simulink library "libbha_parameters"  (R2015b)
settings: Solver=FixedStepDiscrete  StartTime=0.0  StopTime=Inf  FixedStep=0.004  RelTol=1e-3
PostLoadFcn:
  | , if any(exist('dsrtsu_mdlpostloadfcn', 'file') == [2, 3, 6]), try dsrtsu_mdlpostloadfcn('Execute', bdroot); catch fprintf('Error in PostLoadFcn (dsrtsu_mdlpostloadfcn) for model "%s":\n %s\n', bdroot, lasterr); end, end,
undefined symbols (not defined in the file or in its folder): BHA, CONST
libraries: libbha_kinematic x12
(part 2 of 2)

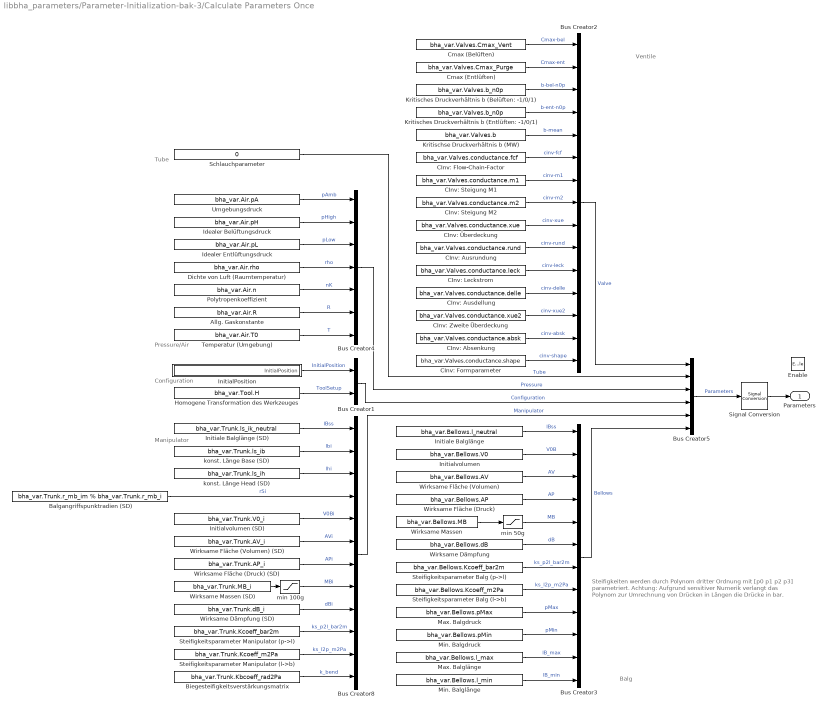
== system libbha_parameters/Parameter-Initialization-bak-3/Calculate Parameters Once ==
  note: Tube
  note: Pressure/Air
  note: Configuration
  note: Manipulator
  note: Ventile
  note: Balg
  note: Steifigkeiten werden durch Polynom dritter Ordnung mit [p0 p1 p2 p3]
      | parametriert. Achtung: Aufgrund sensitiver Numerik verlangt das Polynom
      | zur Umrechnung von Drücken in Längen die Drücke in bar.
  Enable : EnablePort  PropagateVarSize=During execution
  Allg. Gaskonstante : Constant  Value=bha_var.Air.R
  Balgangriffspunktradien (SD) : Constant  Value=bha_var.Trunk.r_mb_im % bha_var.Trunk.r_mb_i
      settings: AttributesFormatString=|
      | Radien Manipulator-Balg
      | r_mb_im: am Sektionskopf
      | r_mb_i:    an Sektionsmitte
  Biegesteifigkeitsverstärkungsmatrix : Constant  Value=bha_var.Trunk.Kbcoeff_rad2Pa
  Bus Creator1 : BusCreator  Inputs=2
  Bus Creator3 : BusCreator  Inputs=12
  Bus Creator4 : BusCreator  Inputs=7
  Bus Creator8 : BusCreator  Inputs=12
  Bus Creator2 : BusCreator  Inputs=15
  Bus Creator5 : BusCreator  Inputs=6
  CInv: Absenkung : Constant  Value=bha_var.Valves.conductance.absk
  CInv: Ausdellung : Constant  Value=bha_var.Valves.conductance.delle
  CInv: Ausrundung : Constant  Value=bha_var.Valves.conductance.rund
  CInv: Flow-Chain-Factor : Constant  Value=bha_var.Valves.conductance.fcf
  CInv: Formparameter : Constant  Value=bha_var.Valves.conductance.shape
  CInv: Leckstrom : Constant  Value=bha_var.Valves.conductance.leck
  CInv: Steigung M1 : Constant  Value=bha_var.Valves.conductance.m1
  CInv: Steigung M2 : Constant  Value=bha_var.Valves.conductance.m2
  CInv: Zweite Überdeckung : Constant  Value=bha_var.Valves.conductance.xue2
  CInv: Überdeckung : Constant  Value=bha_var.Valves.conductance.xue
  Cmax (Belüften) : Constant  Value=bha_var.Valves.Cmax_Vent
  Cmax (Entlüften) : Constant  Value=bha_var.Valves.Cmax_Purge
  Dichte von Luft (Raumtemperatur) : Constant  Value=bha_var.Air.rho
  Homogene Transformation des Werkzeuges : Constant  Value=bha_var.Tool.H
  Idealer Belüftungsdruck : Constant  Value=bha_var.Air.pH
  Idealer Entlüftungsdruck : Constant  Value=bha_var.Air.pL
  InitialPosition : Subsystem
  Initiale Balglänge : Constant  Value=bha_var.Bellows.l_neutral
  Initiale Balglänge (SD) : Constant  Value=bha_var.Trunk.ls_ik_neutral
  Initialvolumen : Constant  Value=bha_var.Bellows.V0
  Initialvolumen (SD) : Constant  Value=bha_var.Trunk.V0_i
  Kritisches Druckverhältnis b (Belüften: -1/0/1) : Constant  Value=bha_var.Valves.b_n0p
  Kritisches Druckverhältnis b (Entlüften: -1/0/1) : Constant  Value=bha_var.Valves.b_n0p
  Kritischse Druckverhältnis b (MW) : Constant  Value=bha_var.Valves.b
  Max. Balgdruck : Constant  Value=bha_var.Bellows.pMax
  Max. Balglänge : Constant  Value=bha_var.Bellows.l_max
  Min. Balgdruck : Constant  Value=bha_var.Bellows.pMin
  Min. Balglänge : Constant  Value=bha_var.Bellows.l_min
  Polytropenkoeffizient : Constant  Value=bha_var.Air.n
  Schlauchparameter : Constant  Value=0
  Signal Conversion : SignalConversion
  Steifigkeitsparameter Balg (l->b) : Constant  Value=bha_var.Bellows.Kcoeff_m2Pa
  Steifigkeitsparameter Balg (p->l) : Constant  Value=bha_var.Bellows.Kcoeff_bar2m
  Steifigkeitsparameter Manipulator (l->b) : Constant  Value=bha_var.Trunk.Kcoeff_m2Pa
  Steifigkeitsparameter Manipulator (p->l) : Constant  Value=bha_var.Trunk.Kcoeff_bar2m
  Temperatur (Umgebung) : Constant  Value=bha_var.Air.T0
  Umgebungsdruck : Constant  Value=bha_var.Air.pA
  Wirksame Dämpfung : Constant  Value=bha_var.Bellows.dB
  Wirksame Dämpfung (SD) : Constant  Value=bha_var.Trunk.dB_i
  Wirksame Fläche (Druck) : Constant  Value=bha_var.Bellows.AP
  Wirksame Fläche (Druck) (SD) : Constant  Value=bha_var.Trunk.AP_i
  Wirksame Fläche (Volumen) : Constant  Value=bha_var.Bellows.AV
  Wirksame Fläche (Volumen) (SD) : Constant  Value=bha_var.Trunk.AV_i
  Wirksame Massen : Constant  Value=bha_var.Bellows.MB
  Wirksame Massen (SD) : Constant  Value=bha_var.Trunk.MB_i
  konst. Länge Base (SD) : Constant  Value=bha_var.Trunk.ls_ib
  konst. Länge Head (SD) : Constant  Value=bha_var.Trunk.ls_ih
  min 100g : Saturate  UpperLimit=inf  LowerLimit=0.1
  min 50g : Saturate  UpperLimit=inf  LowerLimit=0.1
  Parameters : Outport
  wires:
  CInv: Zweite Überdeckung/1 -> Bus Creator2/13  "cinv-xue2"
  CInv: Ausdellung/1 -> Bus Creator2/12  "cinv-delle"
  CInv: Formparameter/1 -> Bus Creator2/15  "cinv-shape"
  CInv: Absenkung/1 -> Bus Creator2/14  "cinv-absk"
  Kritischse Druckverhältnis b (MW)/1 -> Bus Creator2/5  "b-mean"
  Schlauchparameter/1 -> Bus Creator5/2  "Tube"
  Biegesteifigkeitsverstärkungsmatrix/1 -> Bus Creator8/12  "k_bend"
  Steifigkeitsparameter Manipulator (p->l)/1 -> Bus Creator8/10  "ks_p2l_bar2m"
  Steifigkeitsparameter Manipulator (l->b)/1 -> Bus Creator8/11  "ks_l2p_m2Pa"
  Bus Creator5/1 -> Signal Conversion/1  "Parameters"
  Wirksame Massen/1 -> min 50g/1
  Wirksame Massen (SD)/1 -> min 100g/1
  Umgebungsdruck/1 -> Bus Creator4/1  "pAmb"
  Initiale Balglänge/1 -> Bus Creator3/1  "lBss"
  Wirksame Fläche (Druck)/1 -> Bus Creator3/4  "AP"
  Bus Creator8/1 -> Bus Creator5/5  "Manipulator"
  min 100g/1 -> Bus Creator8/8  "MBi"
  Bus Creator3/1 -> Bus Creator5/6  "Bellows"
  Initialvolumen (SD)/1 -> Bus Creator8/5  "V0Bi"
  Wirksame Dämpfung (SD)/1 -> Bus Creator8/9  "dBi"
  Homogene Transformation des Werkzeuges/1 -> Bus Creator1/2  "ToolSetup"
  Wirksame Fläche (Druck) (SD)/1 -> Bus Creator8/7  "APi"
  Wirksame Fläche (Volumen) (SD)/1 -> Bus Creator8/6  "AVi"
  Initialvolumen/1 -> Bus Creator3/2  "V0B"
  Steifigkeitsparameter Balg (p->l)/1 -> Bus Creator3/7  "ks_p2l_bar2m"
  konst. Länge Head (SD)/1 -> Bus Creator8/3  "lhi"
  konst. Länge Base (SD)/1 -> Bus Creator8/2  "lbi"
  Balgangriffspunktradien (SD)/1 -> Bus Creator8/4  "rSi"
  min 50g/1 -> Bus Creator3/5  "MB"
  Wirksame Dämpfung/1 -> Bus Creator3/6  "dB"
  Dichte von Luft (Raumtemperatur)/1 -> Bus Creator4/4  "rho"
  Temperatur (Umgebung)/1 -> Bus Creator4/7  "T"
  Idealer Entlüftungsdruck/1 -> Bus Creator4/3  "pLow"
  Wirksame Fläche (Volumen)/1 -> Bus Creator3/3  "AV"
  Bus Creator2/1 -> Bus Creator5/1  "Valve"
  Polytropenkoeffizient/1 -> Bus Creator4/5  "nK"
  Allg. Gaskonstante/1 -> Bus Creator4/6  "R"
  InitialPosition/1(InitialPosition) -> Bus Creator1/1  "InitialPosition"
  Steifigkeitsparameter Balg (l->b)/1 -> Bus Creator3/8  "ks_l2p_m2Pa"
  Bus Creator4/1 -> Bus Creator5/3  "Pressure"
  Initiale Balglänge (SD)/1 -> Bus Creator8/1  "lBss"
  Bus Creator1/1 -> Bus Creator5/4  "Configuration"
  Signal Conversion/1 -> Parameters/1
  Idealer Belüftungsdruck/1 -> Bus Creator4/2  "pHigh"
  Kritisches Druckverhältnis b (Belüften: -1/0/1)/1 -> Bus Creator2/3  "b-bel-n0p"
  Cmax (Belüften)/1 -> Bus Creator2/1  "Cmax-bel"
  Cmax (Entlüften)/1 -> Bus Creator2/2  "Cmax-ent"
  Kritisches Druckverhältnis b (Entlüften: -1/0/1)/1 -> Bus Creator2/4  "b-ent-n0p"
  CInv: Leckstrom/1 -> Bus Creator2/11  "cinv-leck"
  CInv: Ausrundung/1 -> Bus Creator2/10  "cinv-rund"
  CInv: Überdeckung/1 -> Bus Creator2/9  "cinv-xue"
  CInv: Steigung M2/1 -> Bus Creator2/8  "cinv-m2"
  CInv: Steigung M1/1 -> Bus Creator2/7  "cinv-m1"
  CInv: Flow-Chain-Factor/1 -> Bus Creator2/6  "cinv-fcf"
  Max. Balgdruck/1 -> Bus Creator3/9  "pMax"
  Min. Balgdruck/1 -> Bus Creator3/10  "pMin"
  Max. Balglänge/1 -> Bus Creator3/11  "lB_max"
  Min. Balglänge/1 -> Bus Creator3/12  "lB_min"

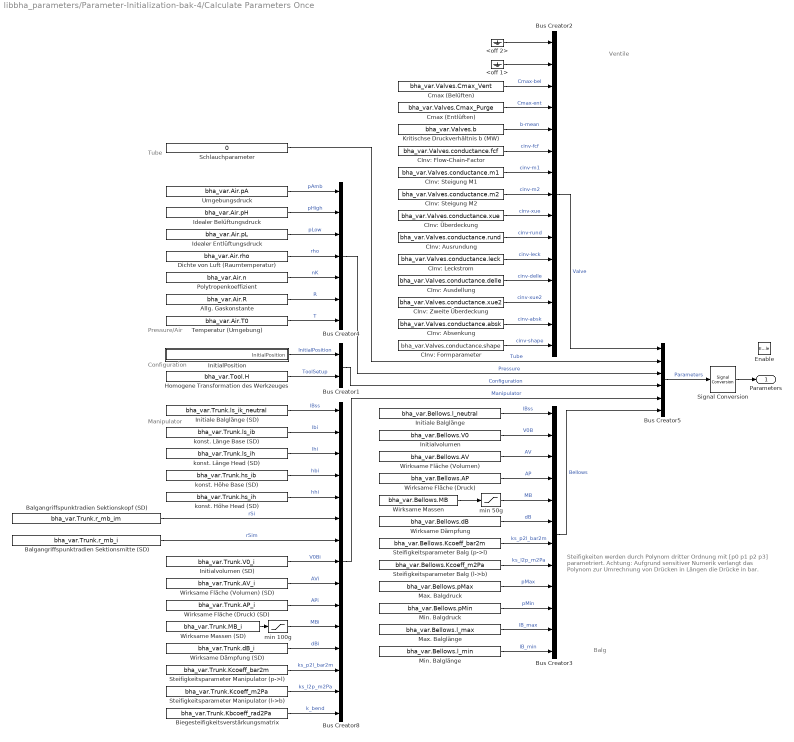
== system libbha_parameters/Parameter-Initialization-bak-4/Calculate Parameters Once ==
  note: Tube
  note: Pressure/Air
  note: Configuration
  note: Manipulator
  note: Ventile
  note: Balg
  note: Steifigkeiten werden durch Polynom dritter Ordnung mit [p0 p1 p2 p3]
      | parametriert. Achtung: Aufgrund sensitiver Numerik verlangt das Polynom
      | zur Umrechnung von Drücken in Längen die Drücke in bar.
  Enable : EnablePort  PropagateVarSize=During execution
  <off 1> : Ground
  <off 2> : Ground
  Allg. Gaskonstante : Constant  Value=bha_var.Air.R
  Balgangriffspunktradien Sektionskopf (SD) : Constant  Value=bha_var.Trunk.r_mb_im
      settings: AttributesFormatString=|
      | Radien Manipulator-Balg
      | r_mb_im: am Sektionskopf
      | r_mb_i:    an Sektionsmitte
      | r_mb_i0:  an Sektionsfuß
  Balgangriffspunktradien Sektionsmitte (SD) : Constant  Value=bha_var.Trunk.r_mb_i
      settings: AttributesFormatString=|
      | Radien Manipulator-Balg
      | r_mb_im: am Sektionskopf
      | r_mb_i:    an Sektionsmitte
      | r_mb_i0:  an Sektionsfuß
  Biegesteifigkeitsverstärkungsmatrix : Constant  Value=bha_var.Trunk.Kbcoeff_rad2Pa
  Bus Creator1 : BusCreator  Inputs=2
  Bus Creator3 : BusCreator  Inputs=12
  Bus Creator4 : BusCreator  Inputs=7
  Bus Creator8 : BusCreator  Inputs=15
  Bus Creator2 : BusCreator  Inputs=15
  Bus Creator5 : BusCreator  Inputs=6
  CInv: Absenkung : Constant  Value=bha_var.Valves.conductance.absk
  CInv: Ausdellung : Constant  Value=bha_var.Valves.conductance.delle
  CInv: Ausrundung : Constant  Value=bha_var.Valves.conductance.rund
  CInv: Flow-Chain-Factor : Constant  Value=bha_var.Valves.conductance.fcf
  CInv: Formparameter : Constant  Value=bha_var.Valves.conductance.shape
  CInv: Leckstrom : Constant  Value=bha_var.Valves.conductance.leck
  CInv: Steigung M1 : Constant  Value=bha_var.Valves.conductance.m1
  CInv: Steigung M2 : Constant  Value=bha_var.Valves.conductance.m2
  CInv: Zweite Überdeckung : Constant  Value=bha_var.Valves.conductance.xue2
  CInv: Überdeckung : Constant  Value=bha_var.Valves.conductance.xue
  Cmax (Belüften) : Constant  Value=bha_var.Valves.Cmax_Vent
  Cmax (Entlüften) : Constant  Value=bha_var.Valves.Cmax_Purge
  Dichte von Luft (Raumtemperatur) : Constant  Value=bha_var.Air.rho
  Homogene Transformation des Werkzeuges : Constant  Value=bha_var.Tool.H
  Idealer Belüftungsdruck : Constant  Value=bha_var.Air.pH
  Idealer Entlüftungsdruck : Constant  Value=bha_var.Air.pL
  InitialPosition : Subsystem
  Initiale Balglänge : Constant  Value=bha_var.Bellows.l_neutral
  Initiale Balglänge (SD) : Constant  Value=bha_var.Trunk.ls_ik_neutral
  Initialvolumen : Constant  Value=bha_var.Bellows.V0
  Initialvolumen (SD) : Constant  Value=bha_var.Trunk.V0_i
  Kritischse Druckverhältnis b (MW) : Constant  Value=bha_var.Valves.b
  Max. Balgdruck : Constant  Value=bha_var.Bellows.pMax
  Max. Balglänge : Constant  Value=bha_var.Bellows.l_max
  Min. Balgdruck : Constant  Value=bha_var.Bellows.pMin
  Min. Balglänge : Constant  Value=bha_var.Bellows.l_min
  Polytropenkoeffizient : Constant  Value=bha_var.Air.n
  Schlauchparameter : Constant  Value=0
  Signal Conversion : SignalConversion
  Steifigkeitsparameter Balg (l->b) : Constant  Value=bha_var.Bellows.Kcoeff_m2Pa
  Steifigkeitsparameter Balg (p->l) : Constant  Value=bha_var.Bellows.Kcoeff_bar2m
  Steifigkeitsparameter Manipulator (l->b) : Constant  Value=bha_var.Trunk.Kcoeff_m2Pa
  Steifigkeitsparameter Manipulator (p->l) : Constant  Value=bha_var.Trunk.Kcoeff_bar2m
  Temperatur (Umgebung) : Constant  Value=bha_var.Air.T0
  Umgebungsdruck : Constant  Value=bha_var.Air.pA
  Wirksame Dämpfung : Constant  Value=bha_var.Bellows.dB
  Wirksame Dämpfung (SD) : Constant  Value=bha_var.Trunk.dB_i
  Wirksame Fläche (Druck) : Constant  Value=bha_var.Bellows.AP
  Wirksame Fläche (Druck) (SD) : Constant  Value=bha_var.Trunk.AP_i
  Wirksame Fläche (Volumen) : Constant  Value=bha_var.Bellows.AV
  Wirksame Fläche (Volumen) (SD) : Constant  Value=bha_var.Trunk.AV_i
  Wirksame Massen : Constant  Value=bha_var.Bellows.MB
  Wirksame Massen (SD) : Constant  Value=bha_var.Trunk.MB_i
  konst. Höhe Base (SD) : Constant  Value=bha_var.Trunk.hs_ib
  konst. Höhe Head (SD) : Constant  Value=bha_var.Trunk.hs_ih
  konst. Länge Base (SD) : Constant  Value=bha_var.Trunk.ls_ib
  konst. Länge Head (SD) : Constant  Value=bha_var.Trunk.ls_ih
  min 100g : Saturate  UpperLimit=inf  LowerLimit=0.1
  min 50g : Saturate  UpperLimit=inf  LowerLimit=0.1
  Parameters : Outport
  wires:
  Biegesteifigkeitsverstärkungsmatrix/1 -> Bus Creator8/15  "k_bend"
  Wirksame Fläche (Volumen) (SD)/1 -> Bus Creator8/9  "AVi"
  Wirksame Fläche (Druck) (SD)/1 -> Bus Creator8/10  "APi"
  Steifigkeitsparameter Manipulator (l->b)/1 -> Bus Creator8/14  "ks_l2p_m2Pa"
  min 100g/1 -> Bus Creator8/11  "MBi"
  Wirksame Dämpfung (SD)/1 -> Bus Creator8/12  "dBi"
  Steifigkeitsparameter Manipulator (p->l)/1 -> Bus Creator8/13  "ks_p2l_bar2m"
  Initialvolumen (SD)/1 -> Bus Creator8/8  "V0Bi"
  Balgangriffspunktradien Sektionsmitte (SD)/1 -> Bus Creator8/7  "rSim"
  Balgangriffspunktradien Sektionskopf (SD)/1 -> Bus Creator8/6  "rSi"
  konst. Höhe Head (SD)/1 -> Bus Creator8/5  "hhi"
  konst. Höhe Base (SD)/1 -> Bus Creator8/4  "hbi"
  <off 2>/1 -> Bus Creator2/1
  <off 1>/1 -> Bus Creator2/2
  CInv: Zweite Überdeckung/1 -> Bus Creator2/13  "cinv-xue2"
  CInv: Ausdellung/1 -> Bus Creator2/12  "cinv-delle"
  CInv: Formparameter/1 -> Bus Creator2/15  "cinv-shape"
  CInv: Absenkung/1 -> Bus Creator2/14  "cinv-absk"
  Kritischse Druckverhältnis b (MW)/1 -> Bus Creator2/5  "b-mean"
  Schlauchparameter/1 -> Bus Creator5/2  "Tube"
  Bus Creator5/1 -> Signal Conversion/1  "Parameters"
  Wirksame Massen/1 -> min 50g/1
  Wirksame Massen (SD)/1 -> min 100g/1
  Umgebungsdruck/1 -> Bus Creator4/1  "pAmb"
  Initiale Balglänge/1 -> Bus Creator3/1  "lBss"
  Wirksame Fläche (Druck)/1 -> Bus Creator3/4  "AP"
  Bus Creator8/1 -> Bus Creator5/5  "Manipulator"
  Bus Creator3/1 -> Bus Creator5/6  "Bellows"
  Homogene Transformation des Werkzeuges/1 -> Bus Creator1/2  "ToolSetup"
  Initialvolumen/1 -> Bus Creator3/2  "V0B"
  Steifigkeitsparameter Balg (p->l)/1 -> Bus Creator3/7  "ks_p2l_bar2m"
  konst. Länge Head (SD)/1 -> Bus Creator8/3  "lhi"
  konst. Länge Base (SD)/1 -> Bus Creator8/2  "lbi"
  min 50g/1 -> Bus Creator3/5  "MB"
  Wirksame Dämpfung/1 -> Bus Creator3/6  "dB"
  Dichte von Luft (Raumtemperatur)/1 -> Bus Creator4/4  "rho"
  Temperatur (Umgebung)/1 -> Bus Creator4/7  "T"
  Idealer Entlüftungsdruck/1 -> Bus Creator4/3  "pLow"
  Wirksame Fläche (Volumen)/1 -> Bus Creator3/3  "AV"
  Bus Creator2/1 -> Bus Creator5/1  "Valve"
  Polytropenkoeffizient/1 -> Bus Creator4/5  "nK"
  Allg. Gaskonstante/1 -> Bus Creator4/6  "R"
  InitialPosition/1(InitialPosition) -> Bus Creator1/1  "InitialPosition"
  Steifigkeitsparameter Balg (l->b)/1 -> Bus Creator3/8  "ks_l2p_m2Pa"
  Bus Creator4/1 -> Bus Creator5/3  "Pressure"
  Initiale Balglänge (SD)/1 -> Bus Creator8/1  "lBss"
  Bus Creator1/1 -> Bus Creator5/4  "Configuration"
  Signal Conversion/1 -> Parameters/1
  Idealer Belüftungsdruck/1 -> Bus Creator4/2  "pHigh"
  Cmax (Belüften)/1 -> Bus Creator2/3  "Cmax-bel"
  Cmax (Entlüften)/1 -> Bus Creator2/4  "Cmax-ent"
  CInv: Leckstrom/1 -> Bus Creator2/11  "cinv-leck"
  CInv: Ausrundung/1 -> Bus Creator2/10  "cinv-rund"
  CInv: Überdeckung/1 -> Bus Creator2/9  "cinv-xue"
  CInv: Steigung M2/1 -> Bus Creator2/8  "cinv-m2"
  CInv: Steigung M1/1 -> Bus Creator2/7  "cinv-m1"
  CInv: Flow-Chain-Factor/1 -> Bus Creator2/6  "cinv-fcf"
  Max. Balgdruck/1 -> Bus Creator3/9  "pMax"
  Min. Balgdruck/1 -> Bus Creator3/10  "pMin"
  Max. Balglänge/1 -> Bus Creator3/11  "lB_max"
  Min. Balglänge/1 -> Bus Creator3/12  "lB_min"

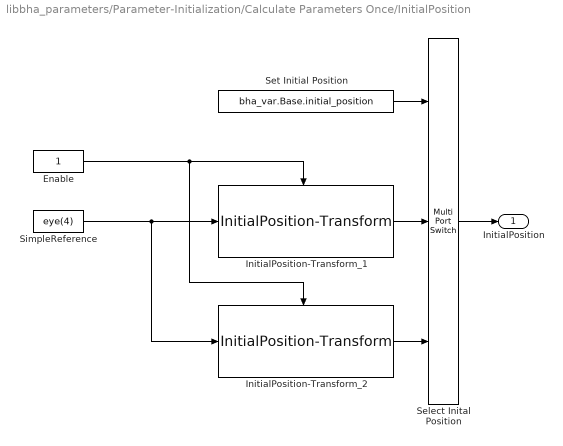
== system libbha_parameters/Parameter-Initialization/Calculate Parameters Once/InitialPosition ==
  Enable : Constant
  InitialPosition-Transform_1 : libbha_kinematic/InitialPosition-Transform  transx=bha_var.Base.initial_translation(1)  transy=bha_var.Base.initial_translation(2)  transz=bha_var.Base.initial_translation(3)  positioning=Hängend  rotz=bha_var.Base.initial_rotation
  InitialPosition-Transform_2 : libbha_kinematic/InitialPosition-Transform  transx=bha_var.Base.initial_translation(1)  transy=bha_var.Base.initial_translation(2)  transz=bha_var.Base.initial_translation(3)  positioning=Stehend  rotz=bha_var.Base.initial_rotation
  Select Inital Position : MultiPortSwitch  Inputs=2  DiagnosticForDefault=Warning
  Set Initial Position : Constant  Value=bha_var.Base.initial_position
  SimpleReference : Constant  Value=eye(4)
  InitialPosition : Outport
  wires:
  Enable/1 -> InitialPosition-Transform_1/Enable, InitialPosition-Transform_2/Enable
  InitialPosition-Transform_2/1 -> Select Inital Position/3
  InitialPosition-Transform_1/1 -> Select Inital Position/2
  SimpleReference/1 -> InitialPosition-Transform_1/1, InitialPosition-Transform_2/1
  Set Initial Position/1 -> Select Inital Position/1
  Select Inital Position/1 -> InitialPosition/1

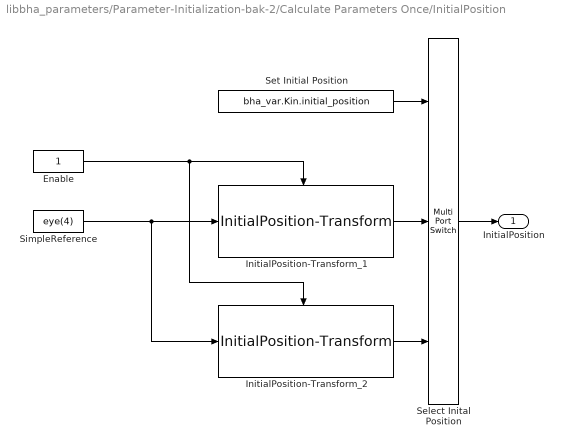
== system libbha_parameters/Parameter-Initialization-bak-2/Calculate Parameters Once/InitialPosition ==
  Enable : Constant
  InitialPosition-Transform_1 : libbha_kinematic/InitialPosition-Transform  transx=bha_var.Kin.initial_translation(1)  transy=bha_var.Kin.initial_translation(2)  transz=bha_var.Kin.initial_translation(3)  positioning=Hängend  rotz=bha_var.Kin.initial_rotation
  InitialPosition-Transform_2 : libbha_kinematic/InitialPosition-Transform  transx=bha_var.Kin.initial_translation(1)  transy=bha_var.Kin.initial_translation(2)  transz=bha_var.Kin.initial_translation(3)  positioning=Stehend  rotz=bha_var.Kin.initial_rotation
  Select Inital Position : MultiPortSwitch  Inputs=2  DiagnosticForDefault=Warning
  Set Initial Position : Constant  Value=bha_var.Kin.initial_position
  SimpleReference : Constant  Value=eye(4)
  InitialPosition : Outport
  wires:
  Select Inital Position/1 -> InitialPosition/1
  Set Initial Position/1 -> Select Inital Position/1
  SimpleReference/1 -> InitialPosition-Transform_2/1, InitialPosition-Transform_1/1
  InitialPosition-Transform_1/1 -> Select Inital Position/2
  InitialPosition-Transform_2/1 -> Select Inital Position/3
  Enable/1 -> InitialPosition-Transform_2/Enable, InitialPosition-Transform_1/Enable

== system libbha_parameters/Parameter-Initialization-bak-2/Calculate Parameters Once/ToolSetup ==
  Enable : Constant  Value=bha_var.Kin.VG_dx
  Enable1 : Constant  Value=bha_var.Kin.VG_dz
  Enable2 : Constant  Value=bha_var.Kin.VG_phiy
  VacuumGripper_Tool : libbha_kinematic/VacuumGripper_Tool
  ToolSetup : Outport
  wires:
  VacuumGripper_Tool/1 -> ToolSetup/1
  Enable/1 -> VacuumGripper_Tool/1
  Enable2/1 -> VacuumGripper_Tool/3
  Enable1/1 -> VacuumGripper_Tool/2

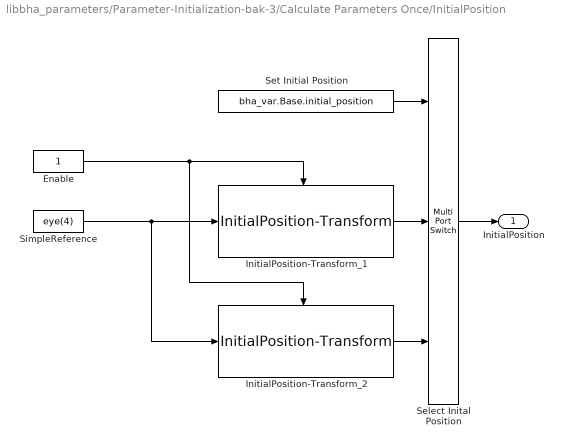
== system libbha_parameters/Parameter-Initialization-bak-3/Calculate Parameters Once/InitialPosition ==
  Enable : Constant
  InitialPosition-Transform_1 : libbha_kinematic/InitialPosition-Transform  transx=bha_var.Base.initial_translation(1)  transy=bha_var.Base.initial_translation(2)  transz=bha_var.Base.initial_translation(3)  positioning=Hängend  rotz=bha_var.Base.initial_rotation
  InitialPosition-Transform_2 : libbha_kinematic/InitialPosition-Transform  transx=bha_var.Base.initial_translation(1)  transy=bha_var.Base.initial_translation(2)  transz=bha_var.Base.initial_translation(3)  positioning=Stehend  rotz=bha_var.Base.initial_rotation
  Select Inital Position : MultiPortSwitch  Inputs=2  DiagnosticForDefault=Warning
  Set Initial Position : Constant  Value=bha_var.Base.initial_position
  SimpleReference : Constant  Value=eye(4)
  InitialPosition : Outport
  wires:
  Select Inital Position/1 -> InitialPosition/1
  Set Initial Position/1 -> Select Inital Position/1
  SimpleReference/1 -> InitialPosition-Transform_2/1, InitialPosition-Transform_1/1
  InitialPosition-Transform_1/1 -> Select Inital Position/2
  InitialPosition-Transform_2/1 -> Select Inital Position/3
  Enable/1 -> InitialPosition-Transform_2/Enable, InitialPosition-Transform_1/Enable

== system libbha_parameters/Parameter-Initialization-bak-4/Calculate Parameters Once/InitialPosition ==
  Enable : Constant
  InitialPosition-Transform_1 : libbha_kinematic/InitialPosition-Transform  transx=bha_var.Base.initial_translation(1)  transy=bha_var.Base.initial_translation(2)  transz=bha_var.Base.initial_translation(3)  positioning=Hängend  rotz=bha_var.Base.initial_rotation
  InitialPosition-Transform_2 : libbha_kinematic/InitialPosition-Transform  transx=bha_var.Base.initial_translation(1)  transy=bha_var.Base.initial_translation(2)  transz=bha_var.Base.initial_translation(3)  positioning=Stehend  rotz=bha_var.Base.initial_rotation
  Select Inital Position : MultiPortSwitch  Inputs=2  DiagnosticForDefault=Warning
  Set Initial Position : Constant  Value=bha_var.Base.initial_position
  SimpleReference : Constant  Value=eye(4)
  InitialPosition : Outport
  wires:
  Select Inital Position/1 -> InitialPosition/1
  Set Initial Position/1 -> Select Inital Position/1
  SimpleReference/1 -> InitialPosition-Transform_2/1, InitialPosition-Transform_1/1
  InitialPosition-Transform_1/1 -> Select Inital Position/2
  InitialPosition-Transform_2/1 -> Select Inital Position/3
  Enable/1 -> InitialPosition-Transform_2/Enable, InitialPosition-Transform_1/Enable

== matlab function libbha_parameters/Parameter-Initialization-bak-2/Calculate Parameters Once/Initialize LookupTable ==
  data: u output; pfcf input; pm1 input; pm2 input; pxue input; prund input; pleck input; y_14 output; y_45 output
function [u, y_14, y_45] = init_norm(pfcf,pm1,pm2,pxue,prund,pleck)
%#codegen

%% Ordinate: Variable Schrittweite
mxue = pxue;

% Datenpunkte: n = 2*n_grob + n_fein
n_grob =  8;
n_fein = 16;

u=[linspace(-1,-mxue*1.2,n_grob),linspace(-mxue*1.1,pxue*1.1,n_fein),linspace(pxue*1.2,1,n_grob)];

%% Ordinate: Alte, feste Schrittweite
%u=[(-1:0.1:-0.2),(-0.18:0.02:0.18),(0.2:0.1:1.0)];



%% Abszisse: Neue, schnelle Version

mfcf = pfcf;
mm1  = pm1;
mm2  = pm2;
mxue = pxue;
mrund = prund;
mleck = pleck;

pC_ges = ((pm2-pm1)*pxue-pm2-pleck)^(-3) + pfcf^(-3);
mC_ges = ((mm2-mm1)*mxue-mm2-mleck)^(-3) + mfcf^(-3);

y_14 =   ((pm1*  u  + (pm2-pm1)*prund*(tanh(( u-pxue)/prund-1)+1)+pleck) .* ((-pleck/pm1<=u )& ( u<pxue+prund)) + (abs((pm2*  u  + (pm1-pm2)*pxue+pleck).^(-3) + pC_ges )).^(-1/3) .* ( u>=pxue+prund));
y_45 = - ((mm1*(-u) + (mm2-mm1)*mrund*(tanh((-u-mxue)/mrund-1)+1)+mleck) .* ( -mleck/mm1<=-u).*(-u<mxue+mrund)  + (abs((mm2*(-u) + (mm1-mm2)*mxue+mleck).^(-3) + mC_ges )).^(-1/3) .* (-u>=mxue+mrund));

end
